simulink model "SIMULINK_01_NON_PARAMETRIC_IDENTIFICATION"  (R2020a)
settings: Solver=FixedStepAuto  StartTime=0.0  StopTime=10  FixedStep=0.001  RelTol=1e-3
settings Model: Creator=alejandropuerta  LastModifiedBy=USUARIO

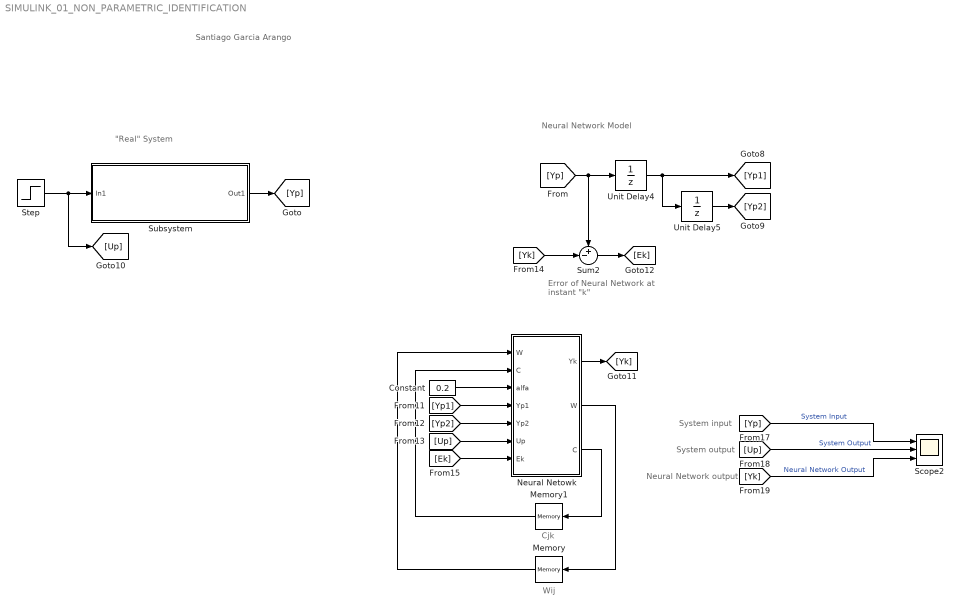
== system SIMULINK_01_NON_PARAMETRIC_IDENTIFICATION ==
  note: Santiago Garcia Arango
  note: Wij
  note: Error of Neural
      | Network at instant "k"
  note: "Real" System
  note: Neural Network Model
  note: Cjk
  note: System input
  note: System output
  note: Neural Network output
  Constant : Constant  Value=0.2
  Memory : Memory  InitialCondition=randn(10,3)
  Memory1 : Memory  InitialCondition=randn(1,10)
  Neural Netowk : MATLAB Function  TreatAsAtomicUnit=on
  Scope2 : Scope  NumInputPorts=3
  Step : Step  Before=1  After=0  SampleTime=0.001
  Subsystem : Subsystem
  Sum2 : Sum  Inputs=+-|
  Unit Delay4 : UnitDelay  SampleTime=-1  HasFrameUpgradeWarning=on
  Unit Delay5 : UnitDelay  SampleTime=-1  HasFrameUpgradeWarning=on
  wires:
  Subsystem/1(Out1) -> [Yp]
  Step/1 -> [Up], Subsystem/1(In1)
  Unit Delay5/1 -> [Yp2]
  Unit Delay4/1 -> [Yp1], Unit Delay5/1
  [Yp] -> Sum2/1, Unit Delay4/1
  Constant/1 -> Neural Netowk/3(alfa)
  [Yp1] -> Neural Netowk/4(Yp1)
  [Yp2] -> Neural Netowk/5(Yp2)
  Neural Netowk/1(Yk) -> [Yk]
  [Yk] -> Sum2/2
  Sum2/1 -> [Ek]
  [Ek] -> Neural Netowk/7(Ek)
  [Up] -> Neural Netowk/6(Up)
  Neural Netowk/2(W) -> Memory/1
  Neural Netowk/3(C) -> Memory1/1
  Memory1/1 -> Neural Netowk/2("C ")
  Memory/1 -> Neural Netowk/1("W ")
  [Yp] -> Scope2/1  "System Input"
  [Up] -> Scope2/2  "System Output"
  [Yk] -> Scope2/3  "Neural Network Output"

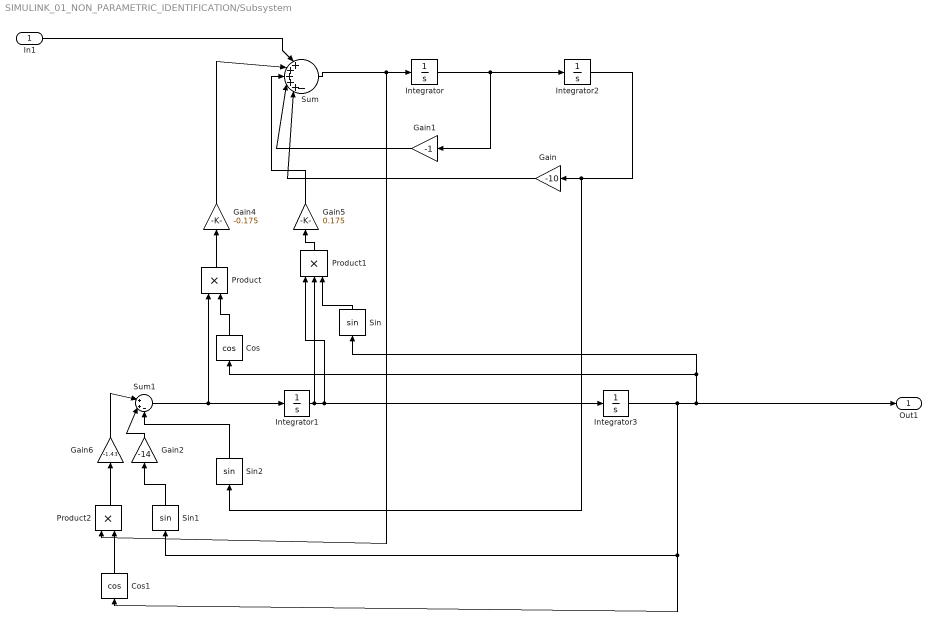
== system SIMULINK_01_NON_PARAMETRIC_IDENTIFICATION/Subsystem ==
  In1 : Inport
  Cos : Trigonometry  Operator=cos
  Cos1 : Trigonometry  Operator=cos
  Gain : Gain  Gain=-10
  Gain1 : Gain  Gain=-1
  Gain2 : Gain  Gain=-14
  Gain4 : Gain  Gain=-0.175
  Gain5 : Gain  Gain=0.175
  Gain6 : Gain  Gain=-1.43
  Integrator{,1..3} (4 alike) : Integrator
  Product : Product
  Product1 : Product  Inputs=3
  Product2 : Product
  Sin : Trigonometry
  Sin1 : Trigonometry
  Sin2 : Trigonometry
  Sum : Sum  Inputs=|+++++-
  Sum1 : Sum  Inputs=|++-
  Out1 : Outport  VectorParamsAs1DForOutWhenUnconnected=off
  wires:
  Integrator/1 -> Gain1/1, Integrator2/1
  Product/1 -> Gain4/1
  Sin/1 -> Product1/3
  Sin1/1 -> Gain2/1
  Product2/1 -> Gain6/1
  Integrator3/1 -> Sin1/1, Cos1/1, Out1/1, Cos/1, Sin/1
  Gain4/1 -> Sum/2
  Sum1/1 -> Product/1, Integrator1/1
  Integrator2/1 -> Sin2/1, Gain/1
  Cos/1 -> Product/2
  Gain5/1 -> Sum/3
  Gain1/1 -> Sum/4
  Product1/1 -> Gain5/1
  Cos1/1 -> Product2/2
  Gain/1 -> Sum/5
  Integrator1/1 -> Integrator3/1, Product1/1, Product1/2
  Gain6/1 -> Sum1/1
  Sum/1 -> Product2/1, Integrator/1
  Sin2/1 -> Sum1/3
  In1/1 -> Sum/1
  Gain2/1 -> Sum1/2

== matlab function SIMULINK_01_NON_PARAMETRIC_IDENTIFICATION/Neural Netowk ==
  data: W input; Yk output; C input; alfa input; Yp1 input; Yp2 input; Up input; Ek input; W output; C output
% NEURAL NETWORK FOR SIMULINK "REAL-TIME" PROCESSING BASED ON SIGNALS
% Santiago Garcia Arango
% ------------------------------------------------------------------------
% FEEDFORWARDMADALINE. Train or Test a simple neural network.
%   alfa: Learning rate constant (1 x 1)
%   W: vector of the initial Weights. size (1 x ne)
%   C: matrix of the initial hidden layers weights. size (ns x no+1)
%   desired: matrix of the desired output, based on entries size (ns x nd)
%   activation_function_x: "none" to pass "Ys" directly.
%   Yp1, Yp2: Original system values (delays)
%   
% ------------------------------------------------------------------------

function [Yk, W, C] = fcn(W, C, alfa, Yp1, Yp2, Up, Ek)

activation_function_1 = "tanh";
activation_function_2 = "none";

X = [Yp1, Yp2, Up]; % Create "entries" vector
Aj = W*X'; % Add hidden layer

if (activation_function_1 == "tanh")
    H = tanh(Aj);
elseif (activation_function_1 == "sigmoidal")
    H = 1./(1 + exp(-Aj));
end


Ak = C'*H; % Add output layer

if (activation_function_2 == "none")
    Yk = Ak;
end

C = C+alfa*Ek*H; % Update weights of C

if (activation_function_1 == "tanh")
    H2 = sech(Aj).^2;
elseif (activation_function_1 == "sigmoidal")
    H2 = H*(1-H);
end

W = W+alfa*Ek*(C.*H2)*X; % Update weights of W
 
end
